simulink model "call_stats_block1"  (R2017b)
settings: Solver=FixedStepAuto  StartTime=0.0  StopTime=10.0  RelTol=1e-3
settings Model: Creator=alic  LastModifiedBy=alic

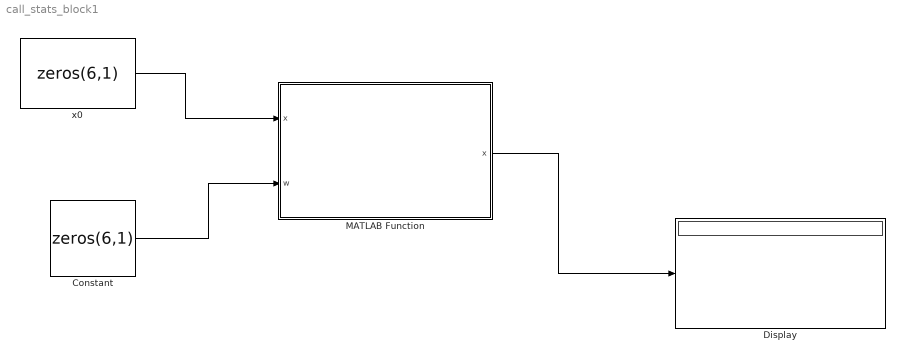
== system call_stats_block1 ==
  Constant : Constant  Value=zeros(6,1)
  Display : Display
  MATLAB Function : MATLAB Function  TreatAsAtomicUnit=on
  x0 : Constant  Value=zeros(6,1)
  wires:
  Constant/1 -> MATLAB Function/2(w)
  x0/1 -> MATLAB Function/1("x ")
  MATLAB Function/1(x) -> Display/1

== matlab function call_stats_block1/MATLAB Function ==
  data: x input; x output; w input
function x = myStateTransitionFcn(x,w)
    %coder.varsize('s');
    %y=zeros(1,2);
    s = zeros(100,6);
    tf = 3;
    t = linspace(0,tf,100);
    [~,s] = ode45(@stateTransition,t, x);
    x = s(100,1:6)';
    % v = s(end,2);
end
